simulink model "sim_sdstd"  (Simulink 6.2)
settings: Solver=ode45  SolverMode=SingleTasking  StartTime=0.0  StopTime=10.0  RelTol=1e-3
undefined symbols (not defined in the file or in its folder): c1, c2, d11, d12, d21, d22, i1, i2, K, n, sys
settings Model: LastModifiedBy=Administrator
settings DataIOCC: SignalLoggingName=sigsOut
settings OptimizationCC: BooleanDataType=off  InlineInvariantSignals=on
settings HardwareCC: TargetUnknown=on

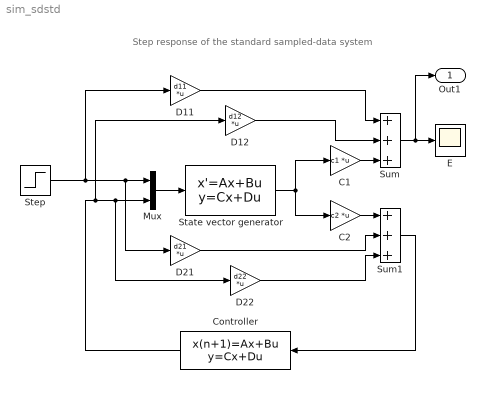
== system sim_sdstd ==
  note: Step response of the standard sampled-data system
  C1 : Gain  Gain=c1  Multiplication=Matrix(K*u)
  C2 : Gain  Gain=c2  Multiplication=Matrix(K*u)
  Controller : DiscreteStateSpace  Orientation=left  A=K.a  B=K.b  C=K.c  D=K.d  SampleTime=K.Ts
  D11 : Gain  Gain=d11  Multiplication=Matrix(K*u)
  D12 : Gain  Gain=d12  Multiplication=Matrix(K*u)
  D21 : Gain  Gain=d21  Multiplication=Matrix(K*u)
  D22 : Gain  Gain=d22  Multiplication=Matrix(K*u)
  E : Scope
      settings: TimeRange=3  YMin=-0.08  YMax=0.09999999999999999  SaveName=SysOut
  Mux : Mux  Inputs=2
  State vector generator : StateSpace  A=sys.a  B=sys.b  C=eye(n)  D=zeros(n,i1+i2)
  Step : Step  Time=0  SampleTime=0
  Sum : Sum  Inputs=+++
  Sum1 : Sum  Inputs=+++
  Out1 : Outport
  wires:
  Mux/1 -> State vector generator/1
  Step/1 -> D11/1, Mux/1, D21/1
  Controller/1 -> D12/1, Mux/2, D22/1
  State vector generator/1 -> C1/1, C2/1
  C1/1 -> Sum/3
  D12/1 -> Sum/2
  D11/1 -> Sum/1
  Sum/1 -> E/1, Out1/1
  C2/1 -> Sum1/1
  D21/1 -> Sum1/2
  D22/1 -> Sum1/3
  Sum1/1 -> Controller/1
